simulink model "C"  (R2023a)
settings: Solver=VariableStepAuto  StartTime=0.0  StopTime=0.1  RelTol=1e-3
libraries: spsSeriesRLCBranchLib x12, spsIGBTDiodeLib x6, spsCurrentMeasurementLib x4, spsVoltageMeasurementLib x4, spsGroundLib x2, spsDCVoltageSourceLib x1, spsMultimeterLib x1, spsThreePhaseVIMeasurementLib x1, sps_lib x1
settings Model: Creator=User  LastModifiedBy=User
settings SolverCC: ZeroCrossAlgorithm=Adaptive
settings DebuggingCC: IgnoredZcDiagnostic=none

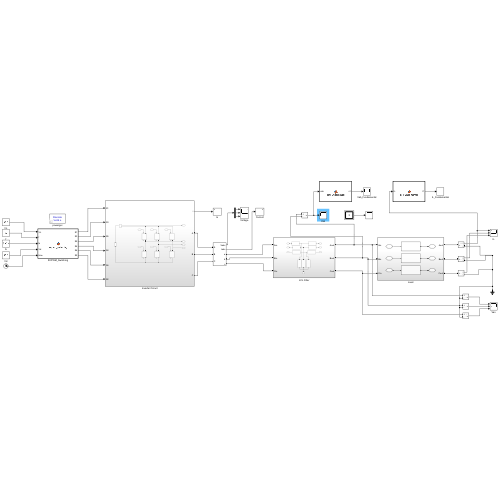
[thumbnail: Simulink's stored preview of the top-level diagram]
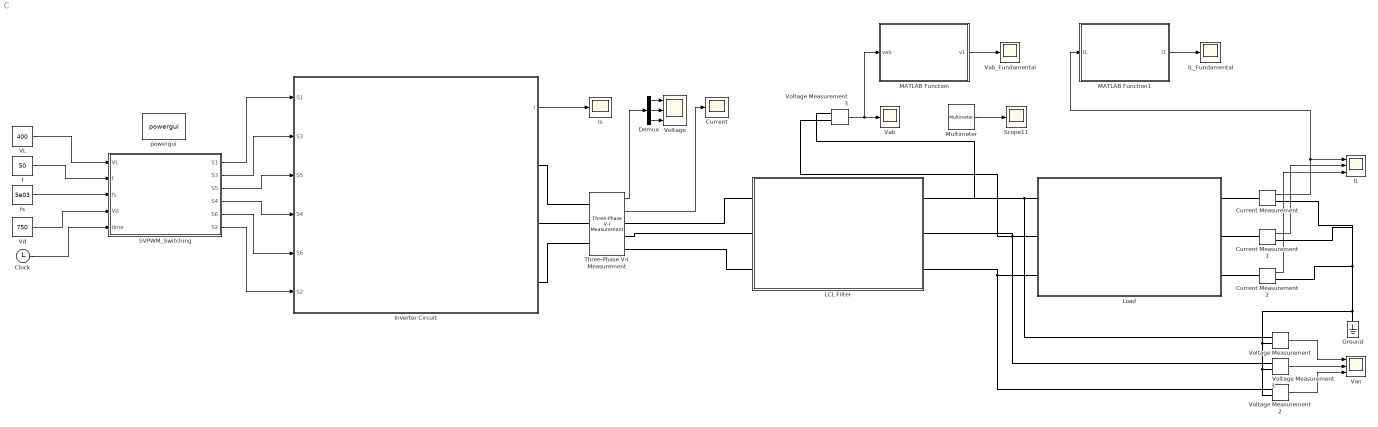
== system C ==
  Clock : Clock
  Current : Scope
  Current Measurement : spsCurrentMeasurementLib/Current Measurement  PhasorSimulation=off  OutputType=Complex  PSBequivalent=0
  Current Measurement1 : spsCurrentMeasurementLib/Current Measurement  PhasorSimulation=off  OutputType=Complex  PSBequivalent=0
  Current Measurement2 : spsCurrentMeasurementLib/Current Measurement  PhasorSimulation=off  OutputType=Complex  PSBequivalent=0
  Demux : Demux  Outputs=3
  Ground : spsGroundLib/Ground  LConnTagsString=a
  IL : Scope  NumInputPorts=3
  IL_Fundamental : Scope
  Inverter Circuit : Subsystem
  Is : Scope
  LCL Filter : Subsystem
  Load : Subsystem
  MATLAB Function : MATLAB Function  TreatAsAtomicUnit=on
  MATLAB Function1 : MATLAB Function  TreatAsAtomicUnit=on
  Multimeter : spsMultimeterLib/Multimeter  L=6  sel=[1 2 3]  yselected={}  Gain=[1 1 1]  OutputType=Complex  PlotAtSimulationStop=off  PhasorSimulation=off
  SVPWM_Switching : MATLAB Function  TreatAsAtomicUnit=on
  Scope11 : Scope
  Three-Phase V-I Measurement : spsThreePhaseVIMeasurementLib/Three-Phase V-I Measurement  VoltageMeasurement=phase-to-phase  SetLabelV=off  LabelV=Vabc  Vpu=off  VpuLL=off  CurrentMeasurement=yes  SetLabelI=off  LabelI=Iabc  Ipu=off  Pbase=100e6  Vbase=500e3  OutputType=Complex  PhasorSimulation=off  PSBequivalent=0
  VL : Constant  Value=400
  Vab : Scope
  Vab_Fundamental : Scope
  Van : Scope  NumInputPorts=3
  Vd : Constant  Value=750
  Voltage : Scope  NumInputPorts=3
  Voltage Measurement{,1..3} (4 alike) : spsVoltageMeasurementLib/Voltage Measurement  PhasorSimulation=off  OutputType=Complex  PSBequivalent=0
  f : Constant  Value=50
  fs : Constant  Value=5e03
  powergui : sps_lib/powergui  Priority=1  SimulationMode=Discrete  SampleTime=10e-7  frequency=60  Iterations=50  frequencyindice=0  Pbase=100e6  ErrMax=1e-4  UnitsV=kV  UnitsW=MW  buscounter=0  FunctionMessages=off  echomessages=off  EnableUseOfTLC=off  CurrentSourceSwitches=off  DisableSnubberDevices=off  DisableRonSwitches=off  DisableVfSwitches=off  DisplayEquations=off  AutomaticDiscreteSolvers=off  SolverType=Tustin/Backward Euler (TBE)  Interpol=off  ExternalGateDelay=off  methode=off  Ts=100  x0status=blocks  SPID=off  SwTol=0  HookPort=off  NonlinearTolerance=1e-4  nMaxIteration=100  ContinueOnMaxIteration=off  RestoreLinks=warning  ResistiveCurrentMeasurement=off  Frange=[0:2:500]  Ylog=off  Xlog=on  ShowGrid=off  save=off  variable=ZData  structure=ScopeData1  ZoomFFT=off  StartTime=0.0  cycles=1  DisplayStyle=1  fundamental=50  FreqAxis=off  MaxFrequency=1000  frequencyindicesteady=1  RmsSteady=1  display=off
  wires:
  Voltage Measurement/1 -> Van/1
  Demux/3 -> Voltage/3
  Demux/1 -> Voltage/1
  Demux/2 -> Voltage/2
  Current Measurement1/1 -> IL/2
  Voltage Measurement2/1 -> Van/3
  Multimeter/1 -> Scope11/1
  Three-Phase V-I Measurement/2 -> Current/1
  Three-Phase V-I Measurement/1 -> Demux/1
  Current Measurement2/1 -> IL/3
  Voltage Measurement1/1 -> Van/2
  Inverter Circuit/1(i) -> Is/1
  SVPWM_Switching/1(S1) -> Inverter Circuit/1(S1)
  SVPWM_Switching/2(S3) -> Inverter Circuit/2(S3)
  SVPWM_Switching/3(S5) -> Inverter Circuit/3(S5)
  SVPWM_Switching/4(S4) -> Inverter Circuit/4(S4)
  SVPWM_Switching/5(S6) -> Inverter Circuit/5(S6)
  SVPWM_Switching/6(S2) -> Inverter Circuit/6(S2)
  Clock/1 -> SVPWM_Switching/5(time)
  Vd/1 -> SVPWM_Switching/4(Vd)
  f/1 -> SVPWM_Switching/2(f)
  VL/1 -> SVPWM_Switching/1(VL)
  fs/1 -> SVPWM_Switching/3(fs)
  Voltage Measurement3/1 -> MATLAB Function/1(vab), Vab/1
  MATLAB Function/1(v1) -> Vab_Fundamental/1
  Current Measurement/1 -> MATLAB Function1/1(IL), IL/1
  MATLAB Function1/1(I1) -> IL_Fundamental/1
  connections:
  Ground/LConn1 -- Current Measurement/RConn1 -- Current Measurement1/RConn1 -- Current Measurement2/RConn1 -- Voltage Measurement2/LConn2 -- Voltage Measurement1/LConn2 -- Voltage Measurement/LConn2
  Voltage Measurement/LConn1 -- Voltage Measurement3/LConn1 -- LCL Filter/RConn1 -- Load/LConn1
  Voltage Measurement1/LConn1 -- Voltage Measurement3/LConn2 -- LCL Filter/RConn2 -- Load/LConn2
  Three-Phase V-I Measurement/LConn1 -- Inverter Circuit/RConn1
  Three-Phase V-I Measurement/LConn2 -- Inverter Circuit/RConn2
  Three-Phase V-I Measurement/LConn3 -- Inverter Circuit/RConn3
  Load/LConn3 -- LCL Filter/RConn3 -- Voltage Measurement2/LConn1
  Current Measurement/LConn1 -- Load/RConn1
  Current Measurement1/LConn1 -- Load/RConn2
  Load/RConn3 -- Current Measurement2/LConn1
  Three-Phase V-I Measurement/RConn1 -- LCL Filter/LConn1
  Three-Phase V-I Measurement/RConn2 -- LCL Filter/LConn2
  Three-Phase V-I Measurement/RConn3 -- LCL Filter/LConn3

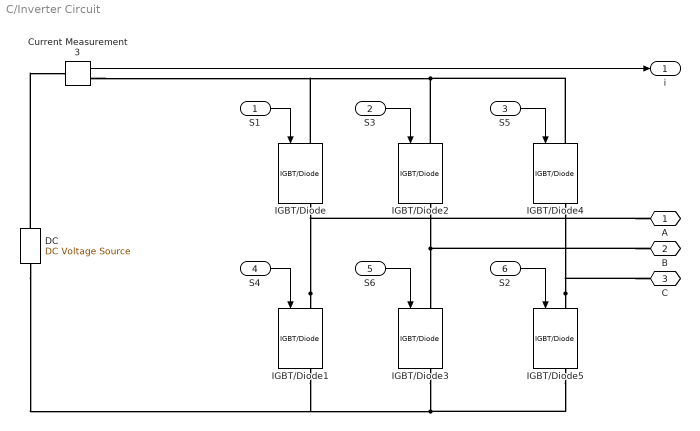
== system C/Inverter Circuit ==
  S1 : Inport
  S3 : Inport  Port=2
  S5 : Inport  Port=3
  S4 : Inport  Port=4
  S6 : Inport  Port=5
  S2 : Inport  Port=6
  Current Measurement3 : spsCurrentMeasurementLib/Current Measurement  PhasorSimulation=off  OutputType=Complex  PSBequivalent=0
  "DC " : spsDCVoltageSourceLib/DC Voltage Source  Amplitude=750  Measurements=None
  IGBT/Diode{,1..5} (6 alike) : spsIGBTDiodeLib/IGBT//Diode  Ron=1e-3  Rs=1e5  Cs=inf  Measurements=on
  A : PMIOPort  Side=Right
  B : PMIOPort  Port=2  Side=Right
  C : PMIOPort  Port=3  Side=Right
  i : Outport
  wires:
  S4/1 -> IGBT/Diode1/1
  S5/1 -> IGBT/Diode4/1
  S1/1 -> IGBT/Diode/1
  Current Measurement3/1 -> i/1
  S2/1 -> IGBT/Diode5/1
  S3/1 -> IGBT/Diode2/1
  S6/1 -> IGBT/Diode3/1
  connections:
  "DC "/RConn1 -- Current Measurement3/LConn1
  IGBT/Diode1/LConn1 -- A/RConn1 -- IGBT/Diode/RConn1
  IGBT/Diode3/RConn1 -- IGBT/Diode5/RConn1 -- IGBT/Diode1/RConn1 -- "DC "/LConn1
  IGBT/Diode2/RConn1 -- IGBT/Diode3/LConn1 -- B/RConn1
  IGBT/Diode2/LConn1 -- IGBT/Diode/LConn1 -- Current Measurement3/RConn1 -- IGBT/Diode4/LConn1
  IGBT/Diode5/LConn1 -- C/RConn1 -- IGBT/Diode4/RConn1

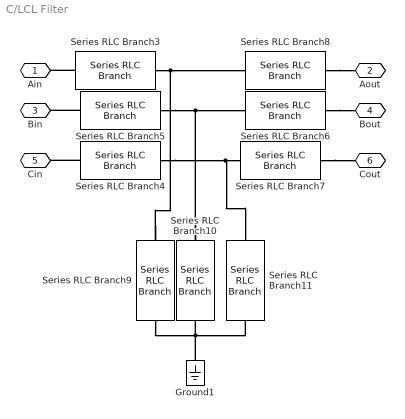
== system C/LCL Filter ==
  Ground1 : spsGroundLib/Ground  LConnTagsString=a
  Series RLC Branch10 : spsSeriesRLCBranchLib/Series RLC Branch  LConnTagsString=__new0  RConnTagsString=__new0  BranchType=C  Resistance=40  Inductance=0.08  SetiL0=off  InitialCurrent=0  Capacitance=150e-6  Setx0=off  InitialVoltage=0  Measurements=None
  Series RLC Branch11 : spsSeriesRLCBranchLib/Series RLC Branch  LConnTagsString=__new0  RConnTagsString=__new0  BranchType=C  Resistance=40  Inductance=0.08  SetiL0=off  InitialCurrent=0  Capacitance=150e-6  Setx0=off  InitialVoltage=0  Measurements=None
  Series RLC Branch{3..8} (6 alike) : spsSeriesRLCBranchLib/Series RLC Branch  LConnTagsString=__new0  RConnTagsString=__new0  BranchType=L  Resistance=40  Inductance=0.03  SetiL0=off  InitialCurrent=0  Capacitance=1e-6  Setx0=off  InitialVoltage=0  Measurements=None
  Series RLC Branch9 : spsSeriesRLCBranchLib/Series RLC Branch  LConnTagsString=__new0  RConnTagsString=__new0  BranchType=C  Resistance=40  Inductance=0.08  SetiL0=off  InitialCurrent=0  Capacitance=150e-6  Setx0=off  InitialVoltage=0  Measurements=None
  Ain : PMIOPort  Side=Left
  Aout : PMIOPort  Port=2  Side=Right
  Bin : PMIOPort  Port=3  Side=Left
  Bout : PMIOPort  Port=4  Side=Right
  Cin : PMIOPort  Port=5  Side=Left
  Cout : PMIOPort  Port=6  Side=Right
  connections:
  Series RLC Branch9/RConn1 -- Series RLC Branch11/RConn1 -- Series RLC Branch10/RConn1 -- Ground1/LConn1
  Series RLC Branch3/LConn1 -- Ain/RConn1
  Series RLC Branch7/RConn1 -- Cout/RConn1
  Series RLC Branch10/LConn1 -- Series RLC Branch6/LConn1 -- Series RLC Branch5/RConn1
  Series RLC Branch7/LConn1 -- Series RLC Branch11/LConn1 -- Series RLC Branch4/RConn1
  Series RLC Branch9/LConn1 -- Series RLC Branch8/LConn1 -- Series RLC Branch3/RConn1
  Series RLC Branch5/LConn1 -- Bin/RConn1
  Series RLC Branch4/LConn1 -- Cin/RConn1
  Series RLC Branch6/RConn1 -- Bout/RConn1
  Series RLC Branch8/RConn1 -- Aout/RConn1

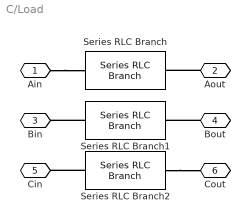
== system C/Load ==
  Series RLC Branch : spsSeriesRLCBranchLib/Series RLC Branch  LConnTagsString=__new0  RConnTagsString=__new0  BranchType=RL  Resistance=40  Inductance=10e-3  SetiL0=off  InitialCurrent=0  Capacitance=1e-6  Setx0=off  InitialVoltage=0  Measurements=Branch voltage and current
  Series RLC Branch1 : spsSeriesRLCBranchLib/Series RLC Branch  LConnTagsString=__new0  RConnTagsString=__new0  BranchType=RL  Resistance=40  Inductance=10e-3  SetiL0=off  InitialCurrent=0  Capacitance=1e-6  Setx0=off  InitialVoltage=0  Measurements=Branch voltage and current
  Series RLC Branch2 : spsSeriesRLCBranchLib/Series RLC Branch  LConnTagsString=__new0  RConnTagsString=__new0  BranchType=RL  Resistance=40  Inductance=10e-3  SetiL0=off  InitialCurrent=0  Capacitance=1e-6  Setx0=off  InitialVoltage=0  Measurements=Branch voltage and current
  Ain : PMIOPort  Side=Left
  Aout : PMIOPort  Port=2  Side=Right
  Bin : PMIOPort  Port=3  Side=Left
  Bout : PMIOPort  Port=4  Side=Right
  Cin : PMIOPort  Port=5  Side=Left
  Cout : PMIOPort  Port=6  Side=Right
  connections:
  Series RLC Branch2/LConn1 -- Cin/RConn1
  Series RLC Branch2/RConn1 -- Cout/RConn1
  Aout/RConn1 -- Series RLC Branch/RConn1
  Series RLC Branch1/LConn1 -- Bin/RConn1
  Ain/RConn1 -- Series RLC Branch/LConn1
  Bout/RConn1 -- Series RLC Branch1/RConn1

== matlab function C/MATLAB Function ==
  data: vab input; v1 output
function v1 = getFundamental(vab)
% Extract 50 Hz fundamental from switching waveform Vab

persistent Ts w A B t As Bs initialized
if isempty(initialized)
    Ts = 1e-6;        % sampling time of your model
    w  = 2*pi*50;     % 50 Hz fundamental
    A  = 0;
    B  = 0;
    t  = 0;
    As = 0;
    Bs = 0;
    initialized = true;
end

% accumulate integrals
A = A + vab * sin(w * t) * Ts;
B = B + vab * cos(w * t) * Ts;

% advance time
t = t + Ts;

% period of 50 Hz
T = 1/50;

% update coefficients every cycle
if t >= T
    As = (2/T) * A;
    Bs = (2/T) * B;

    % reset integrators
    A = 0;
    B = 0;
    t = 0;
end

% reconstruct fundamental voltage
v1 = As * sin(w * t) + Bs * cos(w * t);

== matlab function C/SVPWM_Switching ==
  data: VL input; S1 output; f input; fs input; Vd input; time input; S3 output; S5 output; S4 output; S6 output; S2 output
function [S1, S3, S5, S4, S6, S2] = svpwm_switching(VL, f, fs, Vd, time)
% SVPWM -> Produces gate pulses (0 or 1) for quick testing
% Inputs: VL (rms LL), f (Hz), fs (Hz carrier freq), Vd (DC bus), time (s)
% Outputs: S1,S3,S5 (upper gates), S4,S6,S2 complementary lower gates

Ts = 1/fs;

% ---- Angle ----
theta = mod(360 * f * time, 360);   % degrees
sector = floor(theta/60) + 1; % Sector n ; 1 < n < 6
alpha = deg2rad(theta - (sector-1)*60);

% ---- Modulation index ----
r = (sqrt(6)*VL)/2;
% m = (2*r) / (sqrt(3)*(Vd));   % Vrms->amplitude relation for 3-phase (approx)
m = r / ((sqrt(3)/2) * Vd);
% limit to SVPWM linear region
if m > 0.907
    m = 0.907;
end
if m < 0
    m = 0;
end

% ---- T1, T2, T0 -- center-aligned formula ----
T1 = Ts * m * sin(pi/3 - alpha);
T2 = Ts * m * sin(alpha);
T0 = Ts - T1 - T2;

% avoid negatives
if T1 < 0; T1 = 0; end
if T2 < 0; T2 = 0; end
if T0 < 0; T0 = 0; end

% Pre-init
dA = 0; dB = 0; dC = 0;

% ---- sector duty mapping (centered) ----
switch sector
    case 1
        dA = (T1 + T2 + T0/2)/Ts;
        dB = (T2 + T0/2)/Ts;
        dC = (T0/2)/Ts;
    case 2
        dA = (T1 + T0/2)/Ts;
        dB = (T1 + T2 + T0/2)/Ts;
        dC = (T0/2)/Ts;
    case 3
        dA = (T0/2)/Ts;
        dB = (T1 + T2 + T0/2)/Ts;
        dC = (T2 + T0/2)/Ts;
    case 4
        dA = (T0/2)/Ts;
        dB = (T1 + T0/2)/Ts;
        dC = (T1 + T2 + T0/2)/Ts;
    case 5
        dA = (T2 + T0/2)/Ts;
        dB = (T0/2)/Ts;
        dC = (T1 + T2 + T0/2)/Ts;
    case 6
        dA = (T1 + T2 + T0/2)/Ts;
        dB = (T0/2)/Ts;
        dC = (T1 + T0/2)/Ts;
    otherwise
        dA = 0; dB = 0; dC = 0;
end

% clamp duties to [0,1]
dA = min(max(dA,0),1);
dB = min(max(dB,0),1);
dC = min(max(dC,0),1);

% ---- Carrier phase (sawtooth) 0..1 ----
carrier_phase = mod(time, Ts) / Ts;  % between 0 and 1

% ---- Compare to generate PWM pulses (center-aligned equivalently)
% For center-aligned you might want to compare abs(carrier_phase-0.5) but
% simple leading-edge compare is fine for testing:
S1 = double(carrier_phase < dA);
S3 = double(carrier_phase < dB);
S5 = double(carrier_phase < dC);

% Complementary outputs
S4 = 1 - S1;
S6 = 1 - S3;
S2 = 1 - S5;

end

== matlab function C/MATLAB Function1 ==
  data: IL input; I1 output
function I1 = getFundamental(IL)
% Extract 50 Hz fundamental from switching waveform Vab

persistent Ts w A B t As Bs initialized
if isempty(initialized)
    Ts = 1e-6;        % sampling time of your model
    w  = 2*pi*50;     % 50 Hz fundamental
    A  = 0;
    B  = 0;
    t  = 0;
    As = 0;
    Bs = 0;
    initialized = true;
end

% accumulate integrals
A = A + IL * sin(w * t) * Ts;
B = B + IL * cos(w * t) * Ts;

% advance time
t = t + Ts;

% period of 50 Hz
T = 1/50;

% update coefficients every cycle
if t >= T
    As = (2/T) * A;
    Bs = (2/T) * B;

    % reset integrators
    A = 0;
    B = 0;
    t = 0;
end

% reconstruct fundamental voltage
I1 = As * sin(w * t) + Bs * cos(w * t);
